simulink subsystem "ME591_Power_Cube"  (R2023b)
settings: Solver=VariableStepAuto  StartTime=0.0  StopTime=10.0  RelTol=1e-3
values from neighbouring files (symbols this model uses):
  g0 = 3.173    [project1.m]
libraries: autolibsharedmappedengines x1
(part 2 of 2)

== stateflow chart ME591_Power_Cube/ShiftLogic ==
  settings: sampleTime=0.005
  state gearstate [parallel]
    settings: executionOrder=1
    state first
      gear = 1;
    state second
      gear = 2;
    state third
      gear = 3;
    state fourth
      gear = 4;
    state fifth
      gear = 5;
    state sixth
      gear = 6;
    third -> second [order 1] : down
    fourth -> third [order 1] : down
    fifth -> fourth [order 1] : down
    sixth -> fifth : down
    second -> first [order 1] : down
    (default) -> first
    second -> third [order 2] : up
    third -> fourth [order 2] : up
    fourth -> fifth [order 2] : up
    fifth -> sixth [order 2] : up
    first -> second : up
  state ManualLogic [parallel]
    settings: executionOrder=2
    state steady
      Clutch = 1;
    state clutchup
      Clutch = 0;
    state clutchdown
      Clutch = 0;
    state downshift
      Clutch = 1;
    state upshift
      Clutch = 1;
    (default) -> steady
    steady -> downshift [order 2] : [EngSpd < 1000 && gear>1 ]
    steady -> upshift [order 1] : [EngSpd > 2500 && gear<6]
    downshift -> steady [order 2] : [EngSpd > 1000]
    clutchdown -> steady : after(t_dshift,msec)
        | {send(down,gearstate)}
    upshift -> steady [order 2] : [EngSpd < 2000]
    clutchup -> steady : after(t_upshift,msec)
        | {send(up,gearstate)}
    upshift -> clutchup [order 1] : after(twait,msec)
        | [EngSpd >= 2000]
    downshift -> clutchdown [order 1] : after(twait,msec)
        | [EngSpd <= 1000]
  data: EngSpd input; Clutch output; t_dshift constant double =500; twait constant double =20; t_upshift constant double =500; gear output =1
  events: down local FUNCTION_CALL_EVENT; up local FUNCTION_CALL_EVENT
